simulink model "base_python_example_21a"  (R2021a)
settings: Solver=FixedStepAuto  StartTime=0.0  StopTime=20  FixedStep=0.2  RelTol=1e-3
InitFcn:
  | coeffStds = [0.002995595096857,0.076600147330248,0.631288082601997,0.002600128777275,0.073641936476251,0.984567040148445];
  | coeffMeans = [-1.939450143265110e-04,1.557727430093527e-04,1.473991581706893,-1.909623131136531e-04,0.004474616468621,-1.378729416735388];
  | Isize = single(zeros(227,227));
settings Model: PauseTimes=0.1  Creator=lnarasim  LastModifiedBy=weiwuli
settings SolverCC: AlgebraicLoopSolver=TrustRegion
settings DataIOCC: ReturnWorkspaceOutputs=off
settings DebuggingCC: SFMachineParentedDataDiag=warning  ArithmeticOperatorsInVariantConditions=warning
settings SFSimCC: SimUseLocalCustomCode=off  DefaultCustomCodeFunctionArrayLayout=Row-major  CustomCodeUndefinedFunction=UseInterfaceOnly
settings RTWCC: RTWUseLocalCustomCode=off

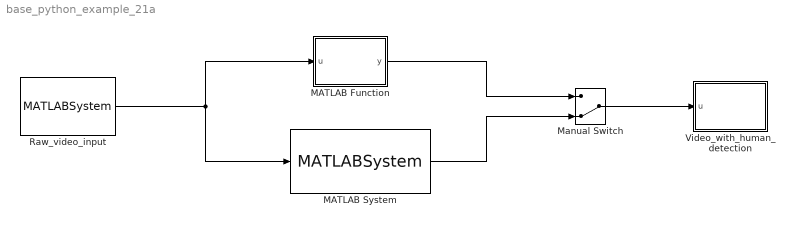
== system base_python_example_21a ==
  MATLAB Function : MATLAB Function  TreatAsAtomicUnit=on
  MATLAB System : MATLABSystem  System=python_HumanDetector  SimulateUsing=Interpreted execution
      mask Type: python_HumanDetector
      mask Display:
      | disp('python_HumanDetector');
      | port_label('input',1,'u');
      | port_label('output',1,'y');
  Manual Switch : ManualSwitch  CurrentSetting=0
  Raw_video_input : MATLABSystem  System=videoReader  SimulateUsing=Interpreted execution
      mask Type: videoReader
      mask Display:
      | disp('videoReader');
      | port_label('output',1,'y');
  Video_with_human_detection : MATLAB Function  TreatAsAtomicUnit=on
  wires:
  MATLAB System/1 -> Manual Switch/2
  MATLAB Function/1(y) -> Manual Switch/1
  Manual Switch/1 -> Video_with_human_detection/1(u)
  Raw_video_input/1 -> MATLAB Function/1(u), MATLAB System/1

== matlab function base_python_example_21a/Video_with_human_detection ==
  data: u input
function fcn(u)
    coder.extrinsic('imagesc');
    imagesc(u);
    drawnow

== matlab function base_python_example_21a/MATLAB Function ==
  data: u input; y output uint8 size=[300, 400, 3]
function y = fcn(u)
    coder.extrinsic('py.detectHuman.getHogObject')
    coder.extrinsic('py.detectHuman.detectHumanFromFrame')
    
    persistent hog;
    if isempty(hog)
        hog = py.detectHuman.getHogObject();
    end
    
    out = py.detectHuman.detectHumanFromFrame(u, hog);
    
    y = uint8(out);
end
